simulink model "signal_test"  (R2019b)
settings: Solver=FixedStepAuto  StartTime=0.0  StopTime=5  FixedStep=0.00001  RelTol=1e-3
undefined symbols (not defined in the file or in its folder): Discrete, Time
libraries: simulink x2, dsparch4 x1, ctrlSharedLib x1, dspstat3 x1
settings Model: Creator=AndreaCalegari  LastModifiedBy=AndreaCalegari

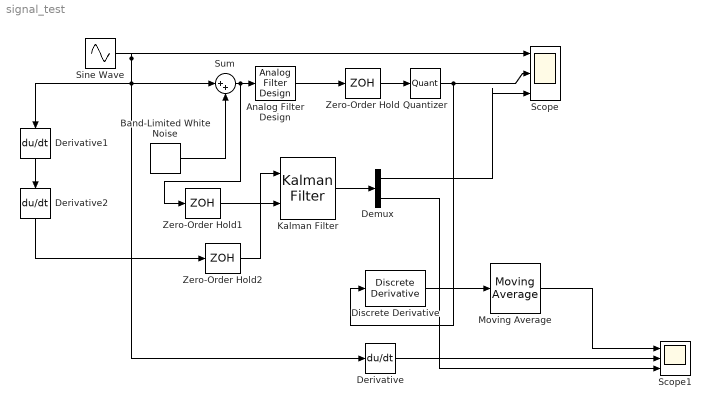
== system signal_test ==
  Analog Filter Design : dsparch4/Analog Filter Design  method=Butterworth  filttype=Lowpass  N=2  Wlo=15  Whi=80  Rp=2  Rs=40
  Band-Limited White Noise : simulink/Sources/Band-Limited White Noise  Cov=[0.00000001]  Ts=0.001  seed=[23341]
  Demux : Demux  Outputs=2
  Derivative : Derivative
  Derivative1 : Derivative
  Derivative2 : Derivative
  Discrete Derivative : simulink/Discrete/Discrete Derivative  gainval=1.0  ICPrevScaledInput=0.0  OutMin=[]  OutMax=[]  OutDataType=fixdt(1, 16)  OutScaling=2^-10  DoSatur=off
  Kalman Filter : ctrlSharedLib/Kalman Filter  TimeDomain=Discrete-Time  UseCurrentEstimator=on  ModelSource=Individual A, B, C, D matrices  ModelSourceVariable=ss(0.95,1,1,0,1)  A=[1,0.00001;0,1]  B=[0;0.00001]  C=[1,0]  D=0  NumberOfStates=1  NumberOfInputs=1  NumberOfOutputs=1  InitialEstimateSource=Dialog  X0=0  P0=10  UseK=off  UseGH=off  NumberOfProcessNoiseInputs=1  G=1  TimeInvariantG=on  H=0  TimeInvariantH=on  Q=0.05  TimeInvariantQ=on  R=0.1  TimeInvariantR=on  N=0  TimeInvariantN=on  AddInputPort=on  AddEnablePort=off  OutputEstimatedY=off  OutputP=off  Ts=-1
      settings: SourceProductBaseCode=CT
  Moving Average : dspstat3/Moving Average  Method=Sliding window  ForgettingFactorPort=off  SpecifyWindowLength=on  WindowLength=500  ForgettingFactor=0.9  SimulateUsing=Code generation
  Quantizer : Quantizer  QuantizationInterval=1/(2^10)
  Scope : Scope  NumInputPorts=3
  Scope1 : Scope  NumInputPorts=3
  Sine Wave : Sin  SampleTime=0
  Sum : Sum  Inputs=|++
  Zero-Order Hold : ZeroOrderHold  SampleTime=-1
  Zero-Order Hold1 : ZeroOrderHold  SampleTime=-1
  Zero-Order Hold2 : ZeroOrderHold  SampleTime=-1
  wires:
  Derivative/1 -> Scope1/2
  Discrete Derivative/1 -> Moving Average/1
  Band-Limited White Noise/1 -> Sum/2
  Sine Wave/1 -> Scope/1, Derivative1/1, Sum/1, Derivative/1
  Zero-Order Hold/1 -> Quantizer/1
  Quantizer/1 -> Scope/2, Discrete Derivative/1
  Moving Average/1 -> Scope1/1
  Sum/1 -> Zero-Order Hold1/1, Analog Filter Design/1
  Analog Filter Design/1 -> Zero-Order Hold/1
  Zero-Order Hold1/1 -> Kalman Filter/2
  Kalman Filter/1 -> Demux/1
  Derivative1/1 -> Derivative2/1
  Derivative2/1 -> Zero-Order Hold2/1
  Zero-Order Hold2/1 -> Kalman Filter/1
  Demux/2 -> Scope1/3
  Demux/1 -> Scope/3
